simulink subsystem "sub_sensor"  (R2023b)
settings: Solver=VariableStepAuto  StartTime=0.0  StopTime=10.0  RelTol=1e-3
libraries: arduinolib x2
settings Model: Creator=ricfe  LastModifiedBy=ricfe

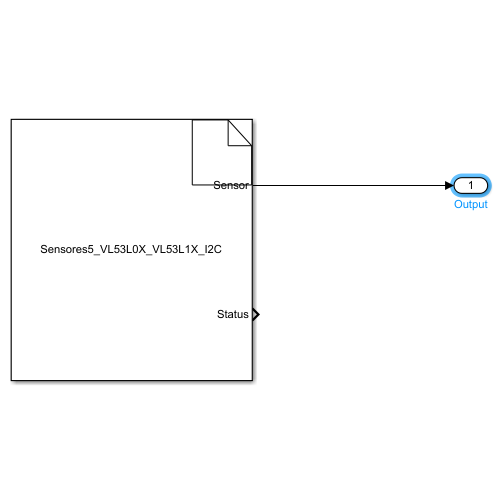
[thumbnail: Simulink's stored preview of the top-level diagram]
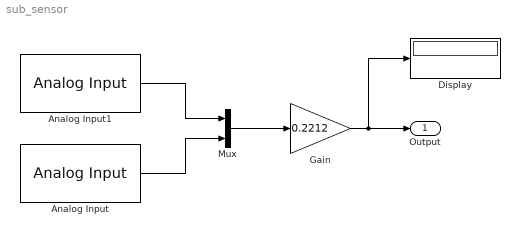
== system sub_sensor ==
  Analog Input : arduinolib/Analog Input  pinNumber=4  ReadResultsOnly=off  ConversionTriggerSource=Software  ExternalTriggerType=uint32( 0 )  OutputDataType=uint16  EnableConversionCompleteNotify=off  EnableOuputStatus=off  SampleTime=-1  blockPlatform=arduino
  Analog Input1 : arduinolib/Analog Input  pinNumber=5  ReadResultsOnly=off  ConversionTriggerSource=Software  ExternalTriggerType=uint32( 0 )  OutputDataType=uint16  EnableConversionCompleteNotify=off  EnableOuputStatus=off  SampleTime=-1  blockPlatform=arduino
  Display : Display
  Gain : Gain  Gain=0.2212  OutDataTypeStr=double
  Mux : Mux  Inputs=2
  Output : Outport
  wires:
  Mux/1 -> Gain/1
  Analog Input/1 -> Mux/2
  Analog Input1/1 -> Mux/1
  Gain/1 -> Output/1, Display/1
